simulink model "EMR_vehicle_model"  (R2023a)
settings: Solver=VariableStepAuto  StartTime=0.0  StopTime=sim_time  RelTol=1e-3
values from neighbouring files (symbols this model uses):
  A_f = 2    [motor_parameters.m]
  air_dens = 1.22521    [motor_parameters.m]
  angle_road = atan(slope_road/100)    [motor_parameters.m]
  C_d = 0.35    [motor_parameters.m]
  emf_constant = 1.2396    [motor_parameters.m]
  f_r = 0.017    [motor_parameters.m]
  g = 9.8    [motor_parameters.m]
  k_gear = 5    [motor_parameters.m]
  Ki_current = (log(9)/risingtime)*winding_resistance    [motor_parameters.m]
  Kp_current = (log(9)/risingtime)*winding_inductance    [motor_parameters.m]
  Kp_speed = m_v/tau_speed    (= 1000)    [motor_parameters.m]
  m_v = 1000    [motor_parameters.m]
  r_w = 0.26    [motor_parameters.m]
  VDC = 48    [motor_parameters.m]
  wind_speed = 0    [motor_parameters.m]
  winding_inductance = 6.5e-3    (= 0.0065)    [motor_parameters.m]
  winding_resistance = 0.35    [motor_parameters.m]
libraries: simulink x1
settings Model: Creator=citcea  LastModifiedBy=citcea

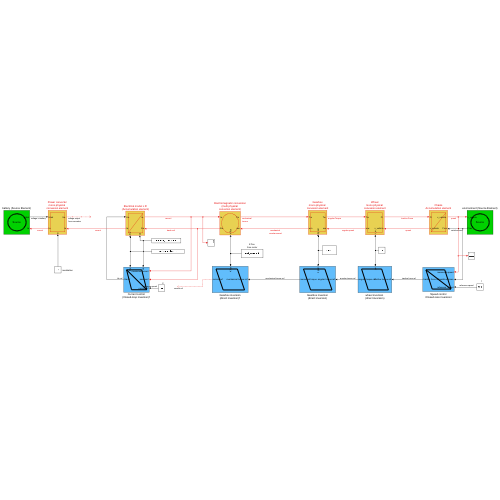
[thumbnail: Simulink's stored preview of the top-level diagram]
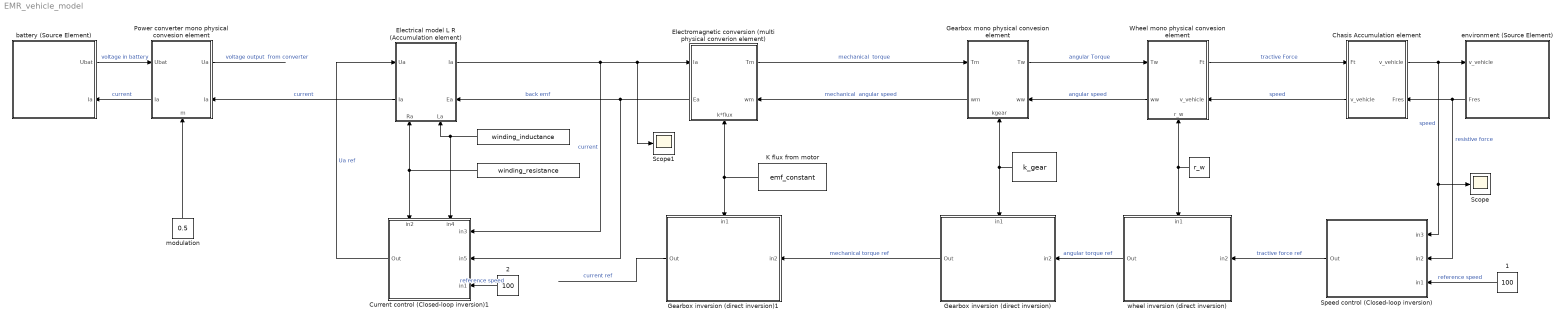
== system EMR_vehicle_model ==
  " " : Constant  Value=winding_resistance
  "  " : Constant  Value=k_gear
  "   " : Constant  Value=winding_inductance
  "     " : Constant  Value=r_w
  "     1" : Constant  Value=100
  "     2" : Constant  Value=100
  Chasis Accumulation element : Subsystem  mask(CM){}
      settings: LibrarySourceBlock=simulink/REM/EA  PortSchema="{\"entries\":[{\"content\":{\"sides\":[{\"content\":{\"connectorIds\":[\"In1\",\"Out2\"]},\"type\":\"ConnectorPlacement.EquallySpacedRectSide\",\"uuid\":\"dba36025-b2f5-41cb-9761-d1287a9766e1\"},{\"content\":{\"connectorIds\":[\"Out1\",\"In2\"],\"side\":\"RIGHT\"},\"type\":\"ConnectorPlacement.EquallySpacedRectSide\",\"uuid\":\"3ae5e504-7b8f-4c00-bc0d-c89eccd87070\"},{\"content\":{\"side\":\"TOP\"},\"type\":\"ConnectorPlacement.EquallySpacedRectSide\",\"uuid\":\"a4c04bb5-f94e-4b5c-882d-2c32a11c6b0c\"}]},\"type\":\"ConnectorPlacement.EquallySpacedConnector\",\"uuid\":\"0c2b765b-f129-495b-87a6-76b6e14d78ec\"}],\"packageUris\":[\"http://schema.mathworks.com/mf0/Connector/R2020b\"],\"version\":\"1.0\"}"
      mask Display: plot(0,0,100,100,[10,10,90,90,10],[90,10,10,90,90], [10,90],[10,90])
  Current control (Closed-loop inversion)1 : Subsystem
      settings: PortSchema="{\"entries\":[{\"content\":{\"sides\":[{\"content\":{\"connectorIds\":[\"In1\",\"In2\",\"In3\"]},\"type\":\"ConnectorPlacement.EquallySpacedRectSide\",\"uuid\":\"a820c906-11c6-4dbb-9e11-805d26fb5422\"},{\"content\":{\"connectorIds\":[\"Out1\"],\"side\":\"RIGHT\"},\"type\":\"ConnectorPlacement.EquallySpacedRectSide\",\"uuid\":\"8d44b67b-b289-4efb-a8eb-49d69967bc3c\"},{\"content\":{\"connectorIds\":[\"In4\",\"In5\"],\"side\":\"TOP\"},\"type\":\"ConnectorPlacement.EquallySpacedRectSide\",\"uuid\":\"c429e5d1-75b0-470c-95b9-fb5fa70bd69e\"}]},\"type\":\"ConnectorPlacement.EquallySpacedConnector\",\"uuid\":\"e797d1a4-5aa6-499a-8fb7-224ebc0ccc8b\"}],\"packageUris\":[\"http://schema.mathworks.com/mf0/Connector/R2020b\"],\"version\":\"1.0\"}"
      settings: LibrarySourceBlock=|
      | simulink/SMC/Asservissement
      | Correcteur IP
      mask Display: plot(0,0,100,100, [10,30,90,70,10,90],[90,10,10,90,90,10])
  Electrical model L R (Accumulation element) : Subsystem  mask(CM){}
      settings: LibrarySourceBlock=simulink/REM/EA  PortSchema="{\"entries\":[{\"content\":{\"sides\":[{\"content\":{\"connectorIds\":[\"In1\",\"Out2\"]},\"type\":\"ConnectorPlacement.EquallySpacedRectSide\",\"uuid\":\"eb47d662-bb9b-4acd-af55-2a228b53d8b6\"},{\"content\":{\"connectorIds\":[\"Out1\",\"In4\"],\"side\":\"RIGHT\"},\"type\":\"ConnectorPlacement.EquallySpacedRectSide\",\"uuid\":\"c961b4fe-0170-40df-8b75-bfc3223dfb7e\"},{\"content\":{\"side\":\"TOP\"},\"type\":\"ConnectorPlacement.EquallySpacedRectSide\",\"uuid\":\"6474a77d-3f02-40ef-ac6e-8688b5dfe053\"},{\"content\":{\"connectorIds\":[\"In2\",\"In3\"],\"side\":\"BOTTOM\"},\"type\":\"ConnectorPlacement.EquallySpacedRectSide\",\"uuid\":\"8508c19b-50ed-4acb-b5ce-1a3d4ba68c03\"}]},\"type\":\"ConnectorPlacement.EquallySpacedConnector\",\"uuid\":\"ed0b028c-df9b-42ff-9675-f2eb8371642a\"}],\"packageUris\":[\"http://schema.mathworks.com/mf0/Connector/R2020b\"],\"version\":\"1.0\"}"
      mask Display: plot(0,0,100,100,[10,10,90,90,10],[90,10,10,90,90], [10,90],[10,90])
  Electromagnetic conversion (multi physical converion element) : Subsystem
      settings: LibrarySourceBlock=simulink/REM/EC EM  PortSchema="{\"entries\":[{\"content\":{\"sides\":[{\"content\":{\"connectorIds\":[\"In1\",\"Out2\"]},\"type\":\"ConnectorPlacement.EquallySpacedRectSide\",\"uuid\":\"eb47d662-bb9b-4acd-af55-2a228b53d8b6\"},{\"content\":{\"connectorIds\":[\"Out1\",\"In3\"],\"side\":\"RIGHT\"},\"type\":\"ConnectorPlacement.EquallySpacedRectSide\",\"uuid\":\"c961b4fe-0170-40df-8b75-bfc3223dfb7e\"},{\"content\":{\"side\":\"TOP\"},\"type\":\"ConnectorPlacement.EquallySpacedRectSide\",\"uuid\":\"6474a77d-3f02-40ef-ac6e-8688b5dfe053\"},{\"content\":{\"connectorIds\":[\"In2\"],\"side\":\"BOTTOM\"},\"type\":\"ConnectorPlacement.EquallySpacedRectSide\",\"uuid\":\"5fa3375e-1c74-4447-9856-dc04d4629517\"}]},\"type\":\"ConnectorPlacement.EquallySpacedConnector\",\"uuid\":\"ed0b028c-df9b-42ff-9675-f2eb8371642a\"}],\"packageUris\":[\"http://schema.mathworks.com/mf0/Connector/R2020b\"],\"version\":\"1.0\"}"
      mask Display: plot(0,0,100,100, 1.4*[50,57.68,60.77,63.08,64.97,66.58,68,69.26,70.4, 	71.42,72.36,78.28,80,78.28,72.36,71.42,70.4, 	69.26,68,66.58,64.97,63.08,60.77,57.68,50,42.32, 	39.23,36.92,35.03,33.42,32,30.74,29.6,28.58, 	27.64,21.72,20,21.72,27.64,28.58,29.6,30.74,32, 	33.42,35.03,36.92,39.23,42.32,50]-20, 1.4*[20,21,22,23,24,25,26,27,28,29,30,40,50,60,70,71,72, 	73,74,75,76,77,78,79,80,79,78,77,76,75,74,73,72, 	71,70,60,50,40,30,29,28,27,26,25,24,23,22,21,20]-20)
  Gearbox mono physical convesion element : Subsystem  mask(Hacheur){}
      settings: LibrarySourceBlock=simulink/REM/EC Elec  PortSchema="{\"entries\":[{\"content\":{\"sides\":[{\"content\":{\"connectorIds\":[\"In1\",\"Out2\"]},\"type\":\"ConnectorPlacement.EquallySpacedRectSide\",\"uuid\":\"add9fadb-0fb4-43ab-a2d0-7727804eb2c0\"},{\"content\":{\"connectorIds\":[\"Out1\",\"In3\"],\"side\":\"RIGHT\"},\"type\":\"ConnectorPlacement.EquallySpacedRectSide\",\"uuid\":\"87b3f5c0-7da9-421a-ae8a-66afee038ab7\"},{\"content\":{\"side\":\"TOP\"},\"type\":\"ConnectorPlacement.EquallySpacedRectSide\",\"uuid\":\"1a4f8f42-25ac-452e-8ff7-6a9f16bc9892\"},{\"content\":{\"connectorIds\":[\"In2\"],\"side\":\"BOTTOM\"},\"type\":\"ConnectorPlacement.EquallySpacedRectSide\",\"uuid\":\"62447f74-8a92-4f32-9436-8aa69c6390a6\"}]},\"type\":\"ConnectorPlacement.EquallySpacedConnector\",\"uuid\":\"bc965109-6171-440e-b0fd-d7c986fb98ff\"}],\"packageUris\":[\"http://schema.mathworks.com/mf0/Connector/R2020b\"],\"version\":\"1.0\"}"
      mask Display: plot(0,0,100,100,[10,10,90,90,10],[90,10,10,90,90])
  Gearbox inversion (direct inversion) : Subsystem
      settings: PortSchema="{\"entries\":[{\"content\":{\"sides\":[{\"content\":{\"connectorIds\":[\"In1\"]},\"type\":\"ConnectorPlacement.EquallySpacedRectSide\",\"uuid\":\"89460601-ef91-4e28-89d9-1739ebd446c6\"},{\"content\":{\"connectorIds\":[\"Out1\"],\"side\":\"RIGHT\"},\"type\":\"ConnectorPlacement.EquallySpacedRectSide\",\"uuid\":\"1ce34b6b-3a45-4c28-907b-ce0af421135c\"},{\"content\":{\"connectorIds\":[\"In2\"],\"side\":\"TOP\"},\"type\":\"ConnectorPlacement.EquallySpacedRectSide\",\"uuid\":\"71132fa1-5c16-4a2a-8ec5-329f0796b3f7\"}]},\"type\":\"ConnectorPlacement.EquallySpacedConnector\",\"uuid\":\"f923a9d4-f6d6-49f7-92ef-115028220a52\"}],\"packageUris\":[\"http://schema.mathworks.com/mf0/Connector/R2020b\"],\"version\":\"1.0\"}"
      settings: LibrarySourceBlock=|
      | simulink/SMC/Inversion EC
      | avec mesure
      mask Display: plot(0,0,100,100,[10,30,90,70,10],[90,10,10,90,90])
  Gearbox inversion (direct inversion)1 : Subsystem
      settings: PortSchema="{\"entries\":[{\"content\":{\"sides\":[{\"content\":{\"connectorIds\":[\"In1\"]},\"type\":\"ConnectorPlacement.EquallySpacedRectSide\",\"uuid\":\"89460601-ef91-4e28-89d9-1739ebd446c6\"},{\"content\":{\"connectorIds\":[\"Out1\"],\"side\":\"RIGHT\"},\"type\":\"ConnectorPlacement.EquallySpacedRectSide\",\"uuid\":\"1ce34b6b-3a45-4c28-907b-ce0af421135c\"},{\"content\":{\"connectorIds\":[\"In2\"],\"side\":\"TOP\"},\"type\":\"ConnectorPlacement.EquallySpacedRectSide\",\"uuid\":\"71132fa1-5c16-4a2a-8ec5-329f0796b3f7\"}]},\"type\":\"ConnectorPlacement.EquallySpacedConnector\",\"uuid\":\"f923a9d4-f6d6-49f7-92ef-115028220a52\"}],\"packageUris\":[\"http://schema.mathworks.com/mf0/Connector/R2020b\"],\"version\":\"1.0\"}"
      settings: LibrarySourceBlock=|
      | simulink/SMC/Inversion EC
      | avec mesure
      mask Display: plot(0,0,100,100,[10,30,90,70,10],[90,10,10,90,90])
  K flux from motor : Constant  Value=emf_constant
  Power converter mono physical convesion element : Subsystem  mask(Hacheur){}
      settings: LibrarySourceBlock=simulink/REM/EC Elec  PortSchema="{\"entries\":[{\"content\":{\"sides\":[{\"content\":{\"connectorIds\":[\"In1\",\"Out2\"]},\"type\":\"ConnectorPlacement.EquallySpacedRectSide\",\"uuid\":\"add9fadb-0fb4-43ab-a2d0-7727804eb2c0\"},{\"content\":{\"connectorIds\":[\"Out1\",\"In3\"],\"side\":\"RIGHT\"},\"type\":\"ConnectorPlacement.EquallySpacedRectSide\",\"uuid\":\"87b3f5c0-7da9-421a-ae8a-66afee038ab7\"},{\"content\":{\"side\":\"TOP\"},\"type\":\"ConnectorPlacement.EquallySpacedRectSide\",\"uuid\":\"1a4f8f42-25ac-452e-8ff7-6a9f16bc9892\"},{\"content\":{\"connectorIds\":[\"In2\"],\"side\":\"BOTTOM\"},\"type\":\"ConnectorPlacement.EquallySpacedRectSide\",\"uuid\":\"62447f74-8a92-4f32-9436-8aa69c6390a6\"}]},\"type\":\"ConnectorPlacement.EquallySpacedConnector\",\"uuid\":\"bc965109-6171-440e-b0fd-d7c986fb98ff\"}],\"packageUris\":[\"http://schema.mathworks.com/mf0/Connector/R2020b\"],\"version\":\"1.0\"}"
      mask Display: plot(0,0,100,100,[10,10,90,90,10],[90,10,10,90,90])
  Scope : Scope
  Scope1 : Scope
  Speed control (Closed-loop inversion) : Subsystem
      settings: LibrarySourceBlock=|
      | simulink/SMC/Asservissement
      | Correcteur IP
      mask Display: plot(0,0,100,100, [10,30,90,70,10,90],[90,10,10,90,90,10])
  Wheel mono physical convesion element : Subsystem  mask(Hacheur){}
      settings: LibrarySourceBlock=simulink/REM/EC Elec  PortSchema="{\"entries\":[{\"content\":{\"sides\":[{\"content\":{\"connectorIds\":[\"In1\",\"Out2\"]},\"type\":\"ConnectorPlacement.EquallySpacedRectSide\",\"uuid\":\"add9fadb-0fb4-43ab-a2d0-7727804eb2c0\"},{\"content\":{\"connectorIds\":[\"Out1\",\"In3\"],\"side\":\"RIGHT\"},\"type\":\"ConnectorPlacement.EquallySpacedRectSide\",\"uuid\":\"87b3f5c0-7da9-421a-ae8a-66afee038ab7\"},{\"content\":{\"side\":\"TOP\"},\"type\":\"ConnectorPlacement.EquallySpacedRectSide\",\"uuid\":\"1a4f8f42-25ac-452e-8ff7-6a9f16bc9892\"},{\"content\":{\"connectorIds\":[\"In2\"],\"side\":\"BOTTOM\"},\"type\":\"ConnectorPlacement.EquallySpacedRectSide\",\"uuid\":\"cb138da9-d7db-4398-93fc-4ebc55a3031f\"}]},\"type\":\"ConnectorPlacement.EquallySpacedConnector\",\"uuid\":\"bc965109-6171-440e-b0fd-d7c986fb98ff\"}],\"packageUris\":[\"http://schema.mathworks.com/mf0/Connector/R2020b\"],\"version\":\"1.0\"}"
      mask Display: plot(0,0,100,100,[10,10,90,90,10],[90,10,10,90,90])
  battery (Source Element) : Subsystem
      settings: LibrarySourceBlock=simulink/REM/SE  PortSchema="{\"entries\":[{\"content\":{\"sides\":[{\"content\":{\"connectorIds\":[\"In1\",\"Out1\"]},\"type\":\"ConnectorPlacement.EquallySpacedRectSide\",\"uuid\":\"5172ac9f-d5c1-4cd8-b96a-59474b42a5b1\"},{\"content\":{\"side\":\"RIGHT\"},\"type\":\"ConnectorPlacement.EquallySpacedRectSide\",\"uuid\":\"2f1e5561-012a-4a4f-9618-a2ea7815b4bb\"},{\"content\":{\"side\":\"TOP\"},\"type\":\"ConnectorPlacement.EquallySpacedRectSide\",\"uuid\":\"04863bbd-e2a6-484f-917f-c8a12d5dbdba\"}]},\"type\":\"ConnectorPlacement.EquallySpacedConnector\",\"uuid\":\"d1a021b9-616a-4321-9b00-fb5e0223e97f\"}],\"packageUris\":[\"http://schema.mathworks.com/mf0/Connector/R2020b\"],\"version\":\"1.0\"}"
      mask Display:
      | plot(0,0,100,100, 1.2*[50,57.68,60.77,63.08,64.97,66.58,68,69.26,70.4, 	71.42,72.36,78.28,80,78.28,72.36,71.42,70.4, 	69.26,68,66.58,64.97,63.08,60.77,57.68,50,42.32, 	39.23,36.92,35.03,33.42,32,30.74,29.6,28.58, 	27.64,21.72,20,21.72,27.64,28.58,29.6,30.74,32, 	33.42,35.03,36.92,39.23,42.32,50]-10, 1.2*[20,21,22,23,24,25,26,27,28,29,30,40,50,60,70,71,72, 	73,74,75,76,77,78,79,80,79,78,77,76,75,74,73,72, 	71,70,60,50,40,30,29,28,27,26,25,24,23,22,21,20]-10)
      | disp('Source')
  environment (Source Element) : Subsystem
      settings: LibrarySourceBlock=simulink/REM/SE  PortSchema="{\"entries\":[{\"content\":{\"sides\":[{\"content\":{\"connectorIds\":[\"In1\",\"Out1\"]},\"type\":\"ConnectorPlacement.EquallySpacedRectSide\",\"uuid\":\"5172ac9f-d5c1-4cd8-b96a-59474b42a5b1\"},{\"content\":{\"side\":\"RIGHT\"},\"type\":\"ConnectorPlacement.EquallySpacedRectSide\",\"uuid\":\"2f1e5561-012a-4a4f-9618-a2ea7815b4bb\"},{\"content\":{\"side\":\"TOP\"},\"type\":\"ConnectorPlacement.EquallySpacedRectSide\",\"uuid\":\"04863bbd-e2a6-484f-917f-c8a12d5dbdba\"}]},\"type\":\"ConnectorPlacement.EquallySpacedConnector\",\"uuid\":\"d1a021b9-616a-4321-9b00-fb5e0223e97f\"}],\"packageUris\":[\"http://schema.mathworks.com/mf0/Connector/R2020b\"],\"version\":\"1.0\"}"
      mask Display:
      | plot(0,0,100,100, 1.2*[50,57.68,60.77,63.08,64.97,66.58,68,69.26,70.4, 	71.42,72.36,78.28,80,78.28,72.36,71.42,70.4, 	69.26,68,66.58,64.97,63.08,60.77,57.68,50,42.32, 	39.23,36.92,35.03,33.42,32,30.74,29.6,28.58, 	27.64,21.72,20,21.72,27.64,28.58,29.6,30.74,32, 	33.42,35.03,36.92,39.23,42.32,50]-10, 1.2*[20,21,22,23,24,25,26,27,28,29,30,40,50,60,70,71,72, 	73,74,75,76,77,78,79,80,79,78,77,76,75,74,73,72, 	71,70,60,50,40,30,29,28,27,26,25,24,23,22,21,20]-10)
      | disp('Source')
  modulation : Constant  Value=0.5
  wheel inversion (direct inversion) : Subsystem
      settings: PortSchema="{\"entries\":[{\"content\":{\"sides\":[{\"content\":{\"connectorIds\":[\"In1\"]},\"type\":\"ConnectorPlacement.EquallySpacedRectSide\",\"uuid\":\"89460601-ef91-4e28-89d9-1739ebd446c6\"},{\"content\":{\"connectorIds\":[\"Out1\"],\"side\":\"RIGHT\"},\"type\":\"ConnectorPlacement.EquallySpacedRectSide\",\"uuid\":\"1ce34b6b-3a45-4c28-907b-ce0af421135c\"},{\"content\":{\"connectorIds\":[\"In2\"],\"side\":\"TOP\"},\"type\":\"ConnectorPlacement.EquallySpacedRectSide\",\"uuid\":\"71132fa1-5c16-4a2a-8ec5-329f0796b3f7\"}]},\"type\":\"ConnectorPlacement.EquallySpacedConnector\",\"uuid\":\"f923a9d4-f6d6-49f7-92ef-115028220a52\"}],\"packageUris\":[\"http://schema.mathworks.com/mf0/Connector/R2020b\"],\"version\":\"1.0\"}"
      settings: LibrarySourceBlock=|
      | simulink/SMC/Inversion EC
      | avec mesure
      mask Display: plot(0,0,100,100,[10,30,90,70,10],[90,10,10,90,90])
  wires:
  Chasis Accumulation element/1("v_vehicle ") -> Scope/1, Speed control (Closed-loop inversion)/1(in3), environment (Source Element)/1(v_vehicle)  "speed"
  environment (Source Element)/1(Fres) -> Speed control (Closed-loop inversion)/2(in2), Chasis Accumulation element/2(Fres)  "resistive force"
  Wheel mono physical convesion element/1("Ft ") -> Chasis Accumulation element/1(Ft)  "tractive Force"
  Chasis Accumulation element/2(v_vehicle) -> Wheel mono physical convesion element/3(v_vehicle)  "speed"
  "     "/1 -> Wheel mono physical convesion element/2(r_w), wheel inversion (direct inversion)/2(in1)
  Gearbox mono physical convesion element/1("Tw ") -> Wheel mono physical convesion element/1(Tw)  "angular Torque"
  Wheel mono physical convesion element/2(ww) -> Gearbox mono physical convesion element/3(ww)  "angular speed"
  "  "/1 -> Gearbox inversion (direct inversion)/2(in1), Gearbox mono physical convesion element/2(kgear)
  Electromagnetic conversion (multi physical converion element)/1("Tm ") -> Gearbox mono physical convesion element/1(Tm)  "mechanical  torque"
  Gearbox mono physical convesion element/2(wm) -> Electromagnetic conversion (multi physical converion element)/3(wm)  "mechanical  angular speed"
  Electrical model L R (Accumulation element)/1("Ia ") -> Current control (Closed-loop inversion)1/1(in3), Scope1/1, Electromagnetic conversion (multi physical converion element)/1(Ia)  "current"
  Electromagnetic conversion (multi physical converion element)/2(Ea) -> Current control (Closed-loop inversion)1/2(in5), Electrical model L R (Accumulation element)/4(Ea)  "back emf"
  Electrical model L R (Accumulation element)/2(Ia) -> Power converter mono physical convesion element/3(Ia)  "current"
  Power converter mono physical convesion element/1("Ua ") -> ?  "voltage output  from converter"
  Power converter mono physical convesion element/2("Ia   ") -> battery (Source Element)/1(Ia)  "current"
  battery (Source Element)/1(Ubat) -> Power converter mono physical convesion element/1(Ubat)  "voltage in battery"
  modulation/1 -> Power converter mono physical convesion element/2(m)
  K flux from motor/1 -> Gearbox inversion (direct inversion)1/2(in1), Electromagnetic conversion (multi physical converion element)/2(k*flux)
  " "/1 -> Electrical model L R (Accumulation element)/2(Ra), Current control (Closed-loop inversion)1/5(in2)
  "   "/1 -> Electrical model L R (Accumulation element)/3(La), Current control (Closed-loop inversion)1/4(in4)
  "     1"/1 -> Speed control (Closed-loop inversion)/3(in1)  "reference speed"
  Speed control (Closed-loop inversion)/1(Out) -> wheel inversion (direct inversion)/1(in2)  "tractive force ref"
  wheel inversion (direct inversion)/1(Out) -> Gearbox inversion (direct inversion)/1(in2)  "angular torque ref"
  Gearbox inversion (direct inversion)/1(Out) -> Gearbox inversion (direct inversion)1/1(in2)  "mechanical torque ref"
  Gearbox inversion (direct inversion)1/1(Out) -> ?  "current ref"
  Current control (Closed-loop inversion)1/1(Out) -> Electrical model L R (Accumulation element)/1(Ua)  "Ua ref"
  "     2"/1 -> Current control (Closed-loop inversion)1/3(in1)  "reference speed"

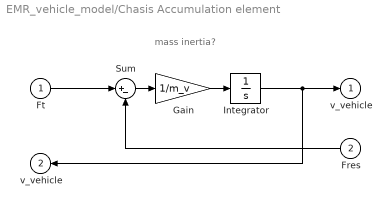
== system EMR_vehicle_model/Chasis Accumulation element ==
  note: mass inertia?
  Ft : Inport
  Fres : Inport  Port=2
  Gain : Gain  Gain=1/m_v
  Integrator : Integrator
  Sum : Sum  Inputs=|+-
  "v_vehicle " : Outport  InitialOutput=0
  v_vehicle : Outport  Port=2  InitialOutput=0
  wires:
  Gain/1 -> Integrator/1
  Sum/1 -> Gain/1
  Integrator/1 -> v_vehicle/1, "v_vehicle "/1
  Ft/1 -> Sum/1
  Fres/1 -> Sum/2

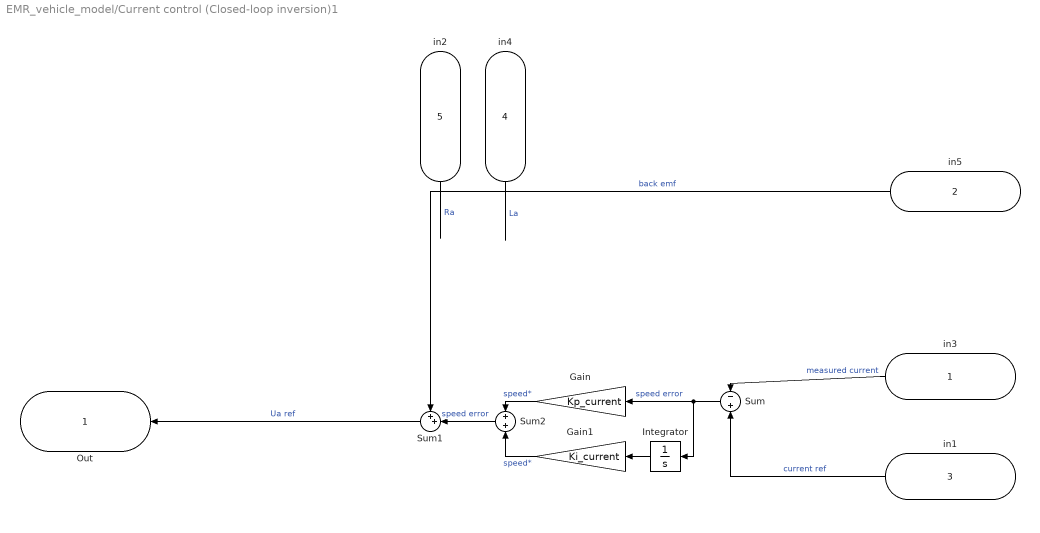
== system EMR_vehicle_model/Current control (Closed-loop inversion)1 ==
  in3 : Inport
  in5 : Inport  Port=2
  in1 : Inport  Port=3
  in4 : Inport  Port=4
  in2 : Inport  Port=5
  Gain : Gain  Gain=Kp_current
  Gain1 : Gain  Gain=Ki_current
  Integrator : Integrator
  Sum : Sum  Inputs=-+
  Sum1 : Sum  Inputs=++|
  Sum2 : Sum
  Out : Outport  InitialOutput=0
  wires:
  in3/1 -> Sum/1  "measured current"
  in1/1 -> Sum/2  "current ref"
  Sum1/1 -> Out/1  "Ua ref"
  Sum/1 -> Integrator/1, Gain/1  "speed error"
  Gain/1 -> Sum2/1  "speed*"
  in2/1 -> ?  "Ra"
  in4/1 -> ?  "La"
  in5/1 -> Sum1/1  "back emf"
  Gain1/1 -> Sum2/2  "speed*"
  Sum2/1 -> Sum1/2  "speed error"
  Integrator/1 -> Gain1/1

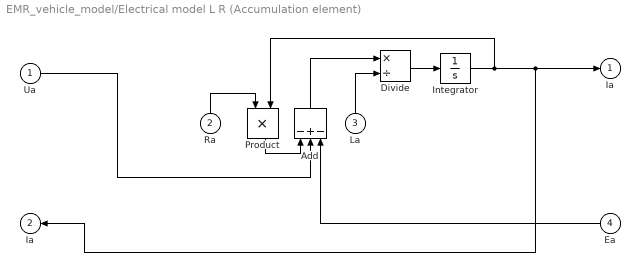
== system EMR_vehicle_model/Electrical model L R (Accumulation element) ==
  Ua : Inport
  Ra : Inport  Port=2
  La : Inport  Port=3
  Ea : Inport  Port=4
  Add : Sum  Inputs=-+-
  Divide : Product  Inputs=*/
  Integrator : Integrator
  Product : Product
  "Ia " : Outport  InitialOutput=0
  Ia : Outport  Port=2  InitialOutput=0
  wires:
  Ea/1 -> Add/3
  Ua/1 -> Add/2
  Integrator/1 -> Product/2, "Ia "/1, Ia/1
  Add/1 -> Divide/1
  La/1 -> Divide/2
  Divide/1 -> Integrator/1
  Product/1 -> Add/1
  Ra/1 -> Product/1

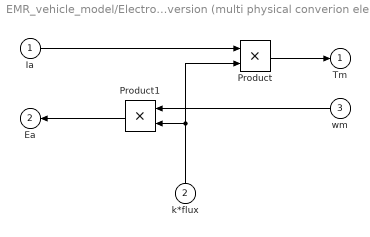
== system EMR_vehicle_model/Electromagnetic conversion (multi physical converion element) ==
  Ia : Inport
  k*flux : Inport  Port=2
  wm : Inport  Port=3
  Product : Product
  Product1 : Product
  "Tm " : Outport  InitialOutput=0
  Ea : Outport  Port=2  InitialOutput=0
  wires:
  Product/1 -> "Tm "/1
  Ia/1 -> Product/1
  k*flux/1 -> Product1/2, Product/2
  Product1/1 -> Ea/1
  wm/1 -> Product1/1

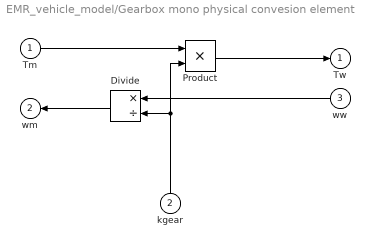
== system EMR_vehicle_model/Gearbox mono physical convesion element ==
  Tm : Inport
  kgear : Inport  Port=2
  ww : Inport  Port=3
  Divide : Product  Inputs=*/
  Product : Product
  "Tw " : Outport  InitialOutput=0
  wm : Outport  Port=2  InitialOutput=0
  wires:
  Divide/1 -> wm/1
  kgear/1 -> Divide/2, Product/2
  ww/1 -> Divide/1
  Product/1 -> "Tw "/1
  Tm/1 -> Product/1

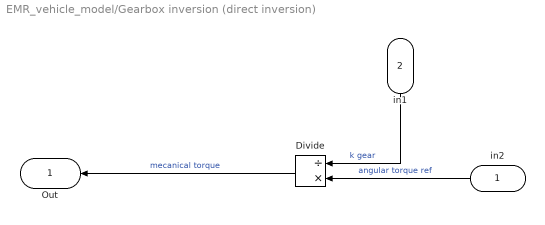
== system EMR_vehicle_model/Gearbox inversion (direct inversion) ==
  in2 : Inport
  in1 : Inport  Port=2
  Divide : Product  Inputs=/*
  Out : Outport  InitialOutput=0
  wires:
  Divide/1 -> Out/1  "mecanical torque"
  in2/1 -> Divide/2  "angular torque ref"
  in1/1 -> Divide/1  "k gear"

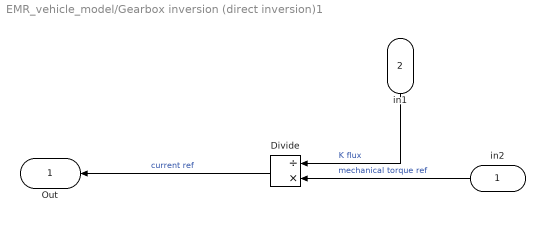
== system EMR_vehicle_model/Gearbox inversion (direct inversion)1 ==
  in2 : Inport
  in1 : Inport  Port=2
  Divide : Product  Inputs=/*
  Out : Outport  InitialOutput=0
  wires:
  in1/1 -> Divide/1  "K flux"
  in2/1 -> Divide/2  "mechanical torque ref"
  Divide/1 -> Out/1  "current ref"

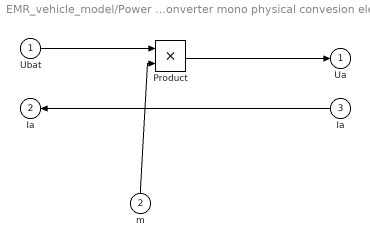
== system EMR_vehicle_model/Power converter mono physical convesion element ==
  Ubat : Inport
  m : Inport  Port=2
  Ia : Inport  Port=3
  Product : Product
  "Ua " : Outport  InitialOutput=0
  "Ia   " : Outport  Port=2  InitialOutput=0
  wires:
  Ia/1 -> "Ia   "/1
  Ubat/1 -> Product/1
  m/1 -> Product/2
  Product/1 -> "Ua "/1

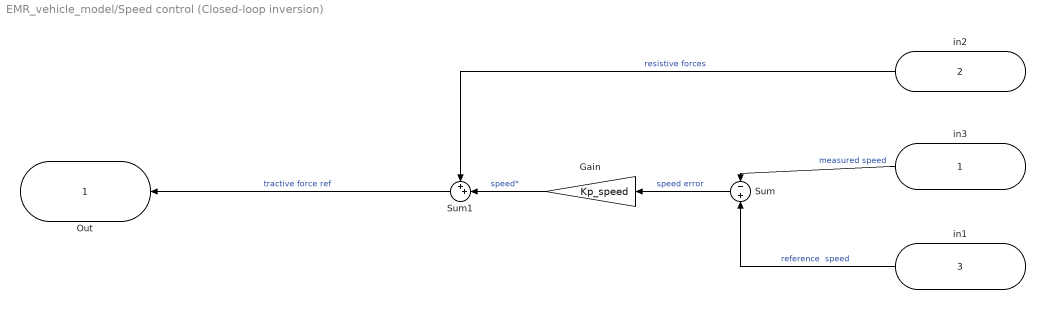
== system EMR_vehicle_model/Speed control (Closed-loop inversion) ==
  in3 : Inport
  in2 : Inport  Port=2
  in1 : Inport  Port=3
  Gain : Gain  Gain=Kp_speed
  Sum : Sum  Inputs=-+
  Sum1 : Sum  Inputs=++|
  Out : Outport  InitialOutput=0
  wires:
  in3/1 -> Sum/1  "measured speed"
  in1/1 -> Sum/2  "reference  speed"
  Sum1/1 -> Out/1  "tractive force ref"
  Sum/1 -> Gain/1  "speed error"
  Gain/1 -> Sum1/2  "speed*"
  in2/1 -> Sum1/1  "resistive forces"

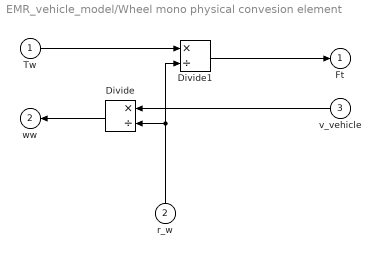
== system EMR_vehicle_model/Wheel mono physical convesion element ==
  Tw : Inport
  r_w : Inport  Port=2
  v_vehicle : Inport  Port=3
  Divide : Product  Inputs=*/
  Divide1 : Product  Inputs=*/
  "Ft " : Outport  InitialOutput=0
  ww : Outport  Port=2  InitialOutput=0
  wires:
  Divide/1 -> ww/1
  v_vehicle/1 -> Divide/1
  r_w/1 -> Divide1/2, Divide/2
  Divide1/1 -> "Ft "/1
  Tw/1 -> Divide1/1

== system EMR_vehicle_model/battery (Source Element) ==
  Ia : Inport
  modulation : Constant  Value=VDC
  Ubat : Outport  InitialOutput=0
  wires:
  modulation/1 -> Ubat/1

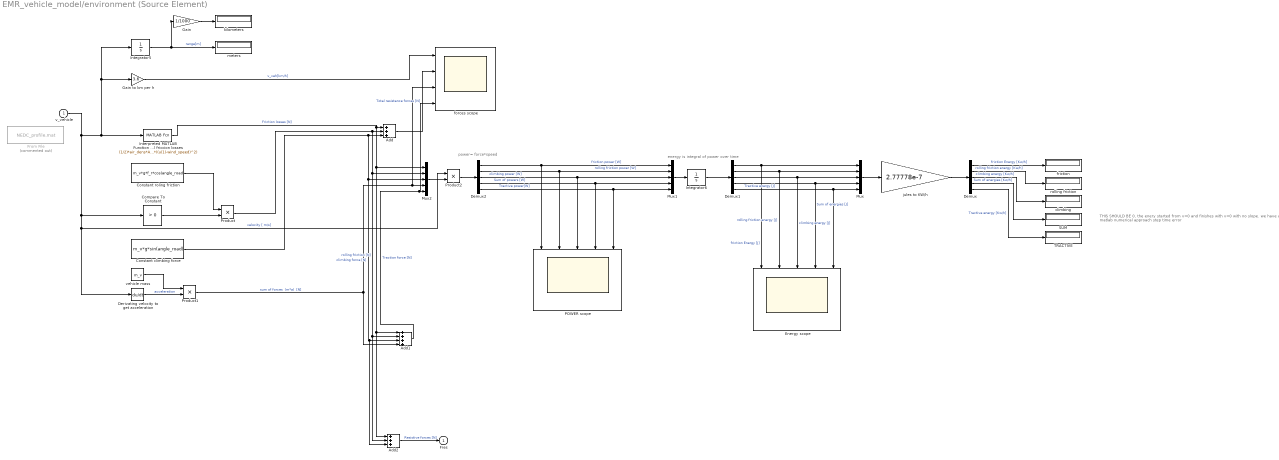
== system EMR_vehicle_model/environment (Source Element) ==
  note: energy is integral of power over time
  note: power= force*speed
  note: THIS SHOULD BE 0, the enery started from v=0 and finishes with v=0 with no slope. we have a matlab numerical approach step time error
  v_vehicle : Inport
  Add : Sum  Inputs=+++
  Add1 : Sum  Inputs=++++
  Add2 : Sum  Inputs=+++
  Compare To Constant : simulink/Logic and Bit Operations/Compare To Constant  relop=>  const=0  OutDataTypeStr=boolean  ZeroCross=off
  Constant climbing force : Constant  Value=m_v*g*sin(angle_road)
  Constant roling friction : Constant  Value=m_v*g*f_r*cos(angle_road)
  Demux : Demux  Outputs=5
  Demux1 : Demux  Outputs=5
  Demux2 : Demux  Outputs=5
  Derivating velocity to get acceleration : Derivative
  Energy scope : Scope  NumInputPorts=5
  From File : FromFile  Commented=on  FileName=NEDC_profile.mat  SampleTime=0
  Gain : Gain  Gain=1/1000
  Gain to km per h : Gain  Gain=3.6
  Integrator5 : Integrator
  Integrator6 : Integrator
  Interpreted MATLAB Function Aerodinamical friccion losses : MATLABFcn  MATLABFcn=(1/2)*air_dens*A_f*C_d*((u(1)-wind_speed)^2)
  Mux : Mux  Inputs=5
  Mux1 : Mux  Inputs=5
  Mux2 : Mux  Inputs=5
  POWER scope : Scope  NumInputPorts=5
  Product : Product
  Product1 : Product
  Product2 : Product
  "SUM " : Display
  TRACTIVE : Display
  climbing : Display
  forces scope : Scope  NumInputPorts=4
  friction : Display
  jules to KW/h : Gain  Gain=2.77778e-7
  kilometers : Display
  meters : Display
  "rolling friction " : Display
  vehicle mass : Constant  Value=m_v
  Fres : Outport  InitialOutput=0
  wires:
  Add2/1 -> Fres/1  "Resistive forces [N]"
  Gain/1 -> kilometers/1
  v_vehicle/1 -> Derivating velocity to get acceleration/1, Product2/1, Compare To Constant/1, Integrator5/1, Gain to km per h/1, Interpreted MATLAB Function Aerodinamical friccion losses/1  "velocity [ m/s]"
  Add1/1 -> forces scope/4, Mux2/5  "Traction force [N]"
  Demux2/2 -> Mux1/2, POWER scope/2  "rolling friction power [W]"
  Integrator5/1 -> Gain/1, meters/1  "range[m]"
  Demux/3 -> climbing/1  "climbing energy [Kw/h]"
  Constant roling friction/1 -> Product/1
  Mux2/1 -> Product2/2
  Gain to km per h/1 -> forces scope/1  "v_veh[km/h]"
  Demux1/3 -> Energy scope/3, Mux/3  "climbing energy [J]"
  Compare To Constant/1 -> Product/2
  Demux2/5 -> Mux1/5, POWER scope/5  "Tractive power[W]"
  Mux1/1 -> Integrator6/1
  Product2/1 -> Demux2/1
  jules to KW/h/1 -> Demux/1
  Demux1/2 -> Energy scope/2, Mux/2  "rolling friction energy [J]"
  Demux/2 -> "rolling friction "/1  "rolling friction energy [Kw/h]"
  Demux2/1 -> Mux1/1, POWER scope/1  "friction power [W]"
  Constant climbing force/1 -> Add2/3, Add1/3, Mux2/3, Add/3  "climbing force [N]"
  Add/1 -> forces scope/2  "Total resistance forces [N]"
  Interpreted MATLAB Function Aerodinamical friccion losses/1 -> Add1/1, Add2/1, Mux2/1, Add/1  "Friction losses [N]"
  Demux2/4 -> Mux1/4, POWER scope/4  "Sum of powers [W]"
  Demux1/4 -> Energy scope/4, Mux/4  "Sum of energies [J]"
  Demux1/1 -> Mux/1, Energy scope/1  "friction Energy [J]"
  Demux1/5 -> Energy scope/5, Mux/5  "Tractive energy [J]"
  Derivating velocity to get acceleration/1 -> Product1/2  "acceleration"
  Integrator6/1 -> Demux1/1
  Mux/1 -> jules to KW/h/1
  Demux2/3 -> Mux1/3, POWER scope/3  "climbing power [W]"
  Product/1 -> Add2/2, Add1/2, Mux2/2, Add/2  "rolling friction [N]"
  Demux/5 -> TRACTIVE/1  "Tractive energy [Kw/h]"
  vehicle mass/1 -> Product1/1
  Demux/4 -> "SUM "/1  "Sum of energies [Kw/h]"
  Demux/1 -> friction/1  "friction Energy [Kw/h]"
  Product1/1 -> Mux2/4, forces scope/3, Add1/4  "sum of forces  (m*a)  [N]"

== system EMR_vehicle_model/wheel inversion (direct inversion) ==
  in2 : Inport
  in1 : Inport  Port=2
  Product : Product
  Out : Outport  InitialOutput=0
  wires:
  Product/1 -> Out/1  "angular torque ref"
  in2/1 -> Product/2  "tractive torque ref"
  in1/1 -> Product/1  "r_w"
